simulink model "cgLQRTest"  (Simulink 7.6)
settings: Solver=ode45  StartTime=0.0  StopTime=10.0  RelTol=1e-3
undefined symbols (not defined in the file or in its folder): cgLQR, CompassGaitPlant, CompassGaitVisualizer
libraries: robotlib x3
settings Model: Creator=russt  LastModifiedBy=russt

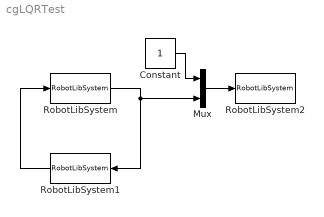
== system cgLQRTest ==
  Constant : Constant
  Mux : Mux  Inputs=2
  RobotLibSystem : robotlib/RobotLibSystem  sysobj=CompassGaitPlant().modes{1}
  RobotLibSystem1 : robotlib/RobotLibSystem  sysobj=cgLQR(CompassGaitPlant().modes{1})
  RobotLibSystem2 : robotlib/RobotLibSystem  sysobj=CompassGaitVisualizer(CompassGaitPlant())
  wires:
  RobotLibSystem/1 -> Mux/2, RobotLibSystem1/1
  RobotLibSystem1/1 -> RobotLibSystem/1
  Mux/1 -> RobotLibSystem2/1
  Constant/1 -> Mux/1
